simulink model "coloumb_bandwitdh"  (R2020a)
settings: Solver=VariableStepAuto  StartTime=0.0  StopTime=100  RelTol=1e-8
values from neighbouring files (symbols this model uses):
  atan_scale = 100    [MandatoryAssignmentB_Loopsyn.m]    (also in MandatoryAssignmentB_Q13.m; MandatoryAssignmentB_Q9.m; threeDiskOscillator_9.m)
  J_1 = 0.0325    [MandatoryAssignmentB_Loopsyn.m]    (also in MandatoryAssignmentB_Q13.m; MandatoryAssignmentB_Q15.m = ECP_values(1); MandatoryAssignmentB_Q9.m = ECP_values(1); threeDiskOscillator_9.m = ECP_values(1))
  T_Cm = ECP_values(13)    [MandatoryAssignmentB_Loopsyn.m]    (also in MandatoryAssignmentB_Q13.m; MandatoryAssignmentB_Q9.m; threeDiskOscillator_9.m)
  T_Cp = ECP_values(12)    [MandatoryAssignmentB_Loopsyn.m]    (also in MandatoryAssignmentB_Q13.m; MandatoryAssignmentB_Q9.m; threeDiskOscillator_9.m)
  w_th = 0.75    [MandatoryAssignmentB_Loopsyn.m]    (also in MandatoryAssignmentB_Q13.m; MandatoryAssignmentB_Q9.m; threeDiskOscillator_9.m)
  x_0 = [0;0;0;0;0;0]    [MandatoryAssignmentB_Q14.m]    (also in MandatoryAssignmentB_Q14_RP.m; MandatoryAssignmentB_Q14_messy.m; MandatoryAssignmentB_Q9.m; threeDiskOscillator_9.m)
settings Model: Creator=dimpa  LastModifiedBy=Administrator
settings DataIOCC: ReturnWorkspaceOutputs=off
settings DebuggingCC: ArithmeticOperatorsInVariantConditions=warning
settings SFSimCC: SimUseLocalCustomCode=off  CustomCodeUndefinedFunction=UseInterfaceOnly
settings RTWCC: RTWUseLocalCustomCode=off

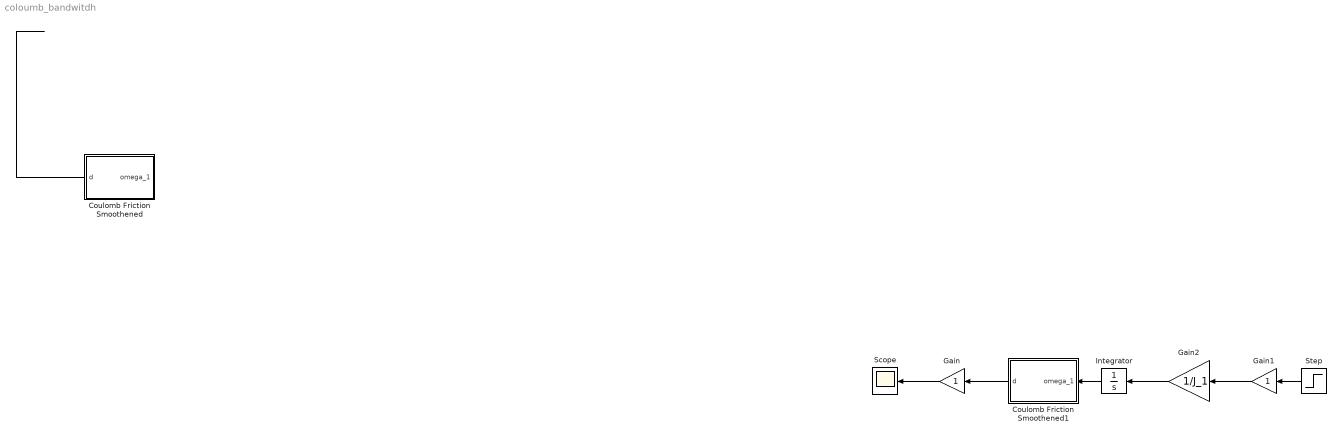
== system coloumb_bandwitdh ==
  Coulomb Friction Smoothened : Subsystem
  Coulomb Friction Smoothened1 : Subsystem
  Gain : Gain
  Gain1 : Gain
  Gain2 : Gain  Gain=1/J_1
  Integrator : Integrator  InitialCondition=x_0(2)
  Scope : Scope
  Step : Step  SampleTime=0
  wires:
  ? -> Coulomb Friction Smoothened/1(omega_1)
  Coulomb Friction Smoothened/1(d) -> ?
  Step/1 -> Gain1/1
  Coulomb Friction Smoothened1/1(d) -> Gain/1
  Gain/1 -> Scope/1
  Gain2/1 -> Integrator/1
  Gain1/1 -> Gain2/1
  Integrator/1 -> Coulomb Friction Smoothened1/1(omega_1)

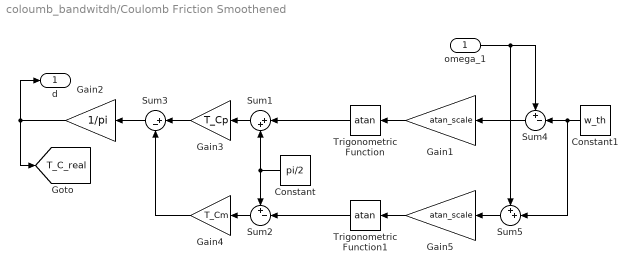
== system coloumb_bandwitdh/Coulomb Friction Smoothened ==
  omega_1 : Inport
  Constant : Constant  Value=pi/2
  Constant1 : Constant  Value=w_th
  Gain1 : Gain  Gain=atan_scale
  Gain2 : Gain  Gain=1/pi
  Gain3 : Gain  Gain=T_Cp
  Gain4 : Gain  Gain=T_Cm
  Gain5 : Gain  Gain=atan_scale
  Sum1 : Sum  Inputs=|++
  Sum2 : Sum  Inputs=+-|
  Sum3 : Sum  Inputs=|+-
  Sum4 : Sum  Inputs=+-|
  Sum5 : Sum  Inputs=++|
  Trigonometric Function : Trigonometry  Operator=atan
  Trigonometric Function1 : Trigonometry  Operator=atan
  d : Outport  VectorParamsAs1DForOutWhenUnconnected=off
  tag scope: T_C_real=global
  wires:
  Gain1/1 -> Trigonometric Function/1
  Sum1/1 -> Gain3/1
  Constant/1 -> Sum2/1, Sum1/2
  Sum2/1 -> Gain4/1
  Sum3/1 -> Gain2/1
  Trigonometric Function/1 -> Sum1/1
  Gain4/1 -> Sum3/2
  Gain2/1 -> [T_C_real], d/1
  omega_1/1 -> Sum5/1, Sum4/1
  Gain3/1 -> Sum3/1
  Sum4/1 -> Gain1/1
  Constant1/1 -> Sum5/2, Sum4/2
  Gain5/1 -> Trigonometric Function1/1
  Sum5/1 -> Gain5/1
  Trigonometric Function1/1 -> Sum2/2

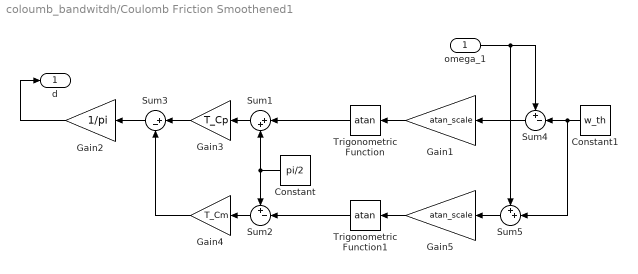
== system coloumb_bandwitdh/Coulomb Friction Smoothened1 ==
  omega_1 : Inport
  Constant : Constant  Value=pi/2
  Constant1 : Constant  Value=w_th
  Gain1 : Gain  Gain=atan_scale
  Gain2 : Gain  Gain=1/pi
  Gain3 : Gain  Gain=T_Cp
  Gain4 : Gain  Gain=T_Cm
  Gain5 : Gain  Gain=atan_scale
  Sum1 : Sum  Inputs=|++
  Sum2 : Sum  Inputs=+-|
  Sum3 : Sum  Inputs=|+-
  Sum4 : Sum  Inputs=+-|
  Sum5 : Sum  Inputs=++|
  Trigonometric Function : Trigonometry  Operator=atan
  Trigonometric Function1 : Trigonometry  Operator=atan
  d : Outport  VectorParamsAs1DForOutWhenUnconnected=off
  wires:
  Gain1/1 -> Trigonometric Function/1
  Sum1/1 -> Gain3/1
  Constant/1 -> Sum2/1, Sum1/2
  Sum2/1 -> Gain4/1
  Sum3/1 -> Gain2/1
  Trigonometric Function/1 -> Sum1/1
  Gain4/1 -> Sum3/2
  Gain2/1 -> d/1
  omega_1/1 -> Sum5/1, Sum4/1
  Gain3/1 -> Sum3/1
  Sum4/1 -> Gain1/1
  Constant1/1 -> Sum5/2, Sum4/2
  Gain5/1 -> Trigonometric Function1/1
  Sum5/1 -> Gain5/1
  Trigonometric Function1/1 -> Sum2/2
